simulink model "study2"  (R2014b)
settings: Solver=ode45  StartTime=0.0  StopTime=10.0  RelTol=1e-3
libraries: powerlib x8
settings Model: Creator=angli  LastModifiedBy=angli

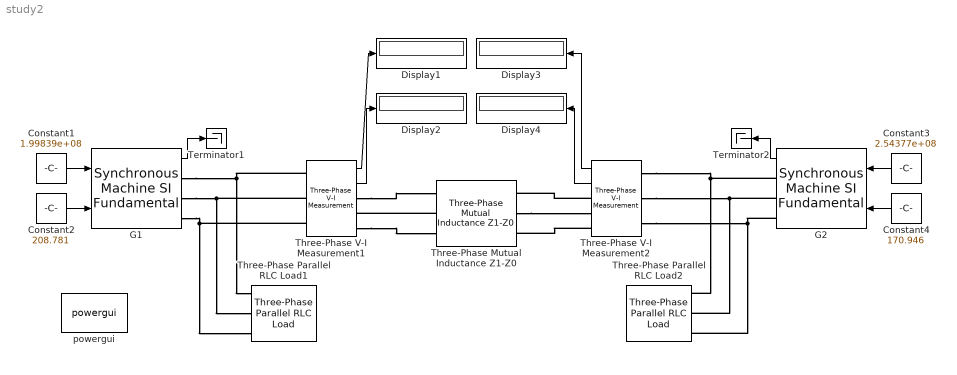
== system study2 ==
  Constant1 : Constant  Value=1.99839e+08
  Constant2 : Constant  Value=208.781
  Constant3 : Constant  Value=2.54377e+08
  Constant4 : Constant  Value=170.946
  Display{1..4} (4 alike) : Display
  G1 : powerlib/Machines/Synchronous Machine SI Fundamental  PresetModel=No  MechanicalLoad=Mechanical power Pm  ShowDetailedParameters=on  RotorType=Salient-pole  Units=SI fundamental parameters  MeasurementBus=off  NominalParameters="[ 100E6  11E3   50   1087 ]"  Stator="[ 2.9069E-03  3.0892E-04  3.2164E-03  9.7153E-04 ]"  Field="[ 5.9013E-04  3.0712E-04 ]"  Dampers2=[ 0.0664, 1.387e-3, 0.0292, 6.896e-4, 7.907e-3, 2.477e-3]  Dampers1="[ 1.1900E-02  4.9076E-04  2.0081E-02  1.0365E-03 ]"  Mechanical=[ 3.895e6 0 20 ]  PolePairs=20  InitialConditions=[0 -101.826 20539.1 20539.1 20539.1 -77.7777 162.222 42.2223 208.781]  SetSaturation=off  Saturation=[695.64,774.7,917.5,1001.6,1082.2,1175.9,1293.6,1430.2,1583.7;9660,10623,12243,13063,13757,14437,15180,15890,16567]  DisplayVfd=off  LoadFlowParameters=[1 198000000 11000 0 0]  TsPowergui=0  TsBlock=-1  IterativeModel=Trapezoidal non iterative  BusType=PV  Pref=0  Qref=0  Qmin=-inf  Qmax=inf  PLF=0  QLF=0
  G2 : powerlib/Machines/Synchronous Machine SI Fundamental  PresetModel=No  MechanicalLoad=Mechanical power Pm  ShowDetailedParameters=on  RotorType=Salient-pole  Units=SI fundamental parameters  MeasurementBus=off  NominalParameters="[ 100E6  11E3   50   1087 ]"  Stator="[ 2.9069E-03  3.0892E-04  3.2164E-03  9.7153E-04 ]"  Field="[ 5.9013E-04  3.0712E-04 ]"  Dampers2=[ 0.0664, 1.387e-3, 0.0292, 6.896e-4, 7.907e-3, 2.477e-3]  Dampers1="[ 1.1900E-02  4.9076E-04  2.0081E-02  1.0365E-03 ]"  Mechanical=[ 3.895e6 0 20 ]  PolePairs=20  InitialConditions=[0 -55.8791 19457.8 19457.8 19457.8 -15.401 -135.401 104.599 170.946]  SetSaturation=off  Saturation=[695.64,774.7,917.5,1001.6,1082.2,1175.9,1293.6,1430.2,1583.7;9660,10623,12243,13063,13757,14437,15180,15890,16567]  DisplayVfd=off  LoadFlowParameters=[2 230000000 0 0 0]  TsPowergui=0  TsBlock=-1  IterativeModel=Trapezoidal non iterative  BusType=PV  Pref=0  Qref=0  Qmin=-inf  Qmax=inf  PLF=0  QLF=0
  Terminator1 : Terminator
  Terminator2 : Terminator
  Three-Phase Mutual Inductance Z1-Z0 : powerlib/Elements/Three-Phase Mutual Inductance Z1-Z0  LConnTagsString=a|b|c  RConnTagsString=A|B|C  PositiveSequence=[2.199780e-01 2.801232e-03]  ZeroSequence=[4.399560e-01 5.602464e-03]
  Three-Phase Parallel RLC Load1 : powerlib/Elements/Three-Phase Parallel RLC Load  LConnTagsString=A|B|C  Configuration=Y (grounded)  NominalVoltage=11E3  NominalFrequency=50  ActivePower=264E6  InductivePower=154E6  CapacitivePower=0  Measurements=None  LoadType=constant Z
  Three-Phase Parallel RLC Load2 : powerlib/Elements/Three-Phase Parallel RLC Load  LConnTagsString=A|B|C  Configuration=Y (grounded)  NominalVoltage=11E3  NominalFrequency=50  ActivePower=176E6  InductivePower=66E6  CapacitivePower=0  Measurements=None  LoadType=constant Z
  Three-Phase V-I Measurement1 : powerlib/Measurements/Three-Phase V-I Measurement  VoltageMeasurement=phase-to-ground  SetLabelV=off  LabelV=Vabc  Vpu=off  VpuLL=off  CurrentMeasurement=yes  SetLabelI=off  LabelI=Iabc  Ipu=off  Pbase=100e6  Vbase=500e3  OutputType=Complex  PhasorSimulation=on  PSBequivalent=0
  Three-Phase V-I Measurement2 : powerlib/Measurements/Three-Phase V-I Measurement  VoltageMeasurement=phase-to-ground  SetLabelV=off  LabelV=Vabc  Vpu=off  VpuLL=off  CurrentMeasurement=yes  SetLabelI=off  LabelI=Iabc  Ipu=off  Pbase=100e6  Vbase=500e3  OutputType=Complex  PhasorSimulation=on  PSBequivalent=0
  powergui : powerlib/powergui  Priority=1  SimulationMode=Phasor  SolverType=Tustin/Backward Euler (TBE)  SampleTime=50e-6  frequency=50  SPID=off  DisableSnubberDevices=off  DisableRonSwitches=off  DisableVfSwitches=off  SwTol=0  DisplayEquations=off  Interpol=off  methode=off  Ts=100  frequencyindice=50  Pbase=100e6  ErrMax=1e-4  Iterations=50  UnitsV=V  UnitsW=W  FunctionMessages=off  echomessages=off  HookPort=off  EnableUseOfTLC=off  x0status=blocks  RestoreLinks=warning  ResistiveCurrentMeasurement=off  Frange=[0:2:500]  Ylog=off  Xlog=on  ShowGrid=off  save=off  variable=ZData  structure=0  ZoomFFT=off  StartTime=0.0  cycles=1  DisplayStyle=1  fundamental=60  FreqAxis=off  MaxFrequency=1000  frequencyindicesteady=1  RmsSteady=1  display=off
  wires:
  G1/1 -> Terminator1/1
  G2/1 -> Terminator2/1
  Constant2/1 -> G1/2
  Constant1/1 -> G1/1
  Constant3/1 -> G2/1
  Constant4/1 -> G2/2
  Three-Phase V-I Measurement1/2 -> Display2/1
  Three-Phase V-I Measurement1/1 -> Display1/1
  Three-Phase V-I Measurement2/1 -> Display3/1
  Three-Phase V-I Measurement2/2 -> Display4/1
  connections:
  G1/RConn1 -- Three-Phase Parallel RLC Load1/LConn1 -- Three-Phase V-I Measurement1/LConn1
  G1/RConn2 -- Three-Phase V-I Measurement1/LConn2 -- Three-Phase Parallel RLC Load1/LConn2
  G1/RConn3 -- Three-Phase Parallel RLC Load1/LConn3 -- Three-Phase V-I Measurement1/LConn3
  G2/RConn1 -- Three-Phase Parallel RLC Load2/LConn1 -- Three-Phase V-I Measurement2/LConn1
  G2/RConn2 -- Three-Phase V-I Measurement2/LConn2 -- Three-Phase Parallel RLC Load2/LConn2
  G2/RConn3 -- Three-Phase V-I Measurement2/LConn3 -- Three-Phase Parallel RLC Load2/LConn3
  Three-Phase Mutual Inductance Z1-Z0/LConn2 -- Three-Phase V-I Measurement1/RConn2
  Three-Phase Mutual Inductance Z1-Z0/RConn2 -- Three-Phase V-I Measurement2/RConn2
  Three-Phase V-I Measurement2/RConn1 -- Three-Phase Mutual Inductance Z1-Z0/RConn1
  Three-Phase V-I Measurement1/RConn1 -- Three-Phase Mutual Inductance Z1-Z0/LConn1
  Three-Phase V-I Measurement1/RConn3 -- Three-Phase Mutual Inductance Z1-Z0/LConn3
  Three-Phase V-I Measurement2/RConn3 -- Three-Phase Mutual Inductance Z1-Z0/RConn3
